simulink model "deadReckoningSim_soln"  (R2017a)
settings: Solver=FixedStepDiscrete  StartTime=0.0  StopTime=15  FixedStep=0.01  RelTol=1e-3
PreLoadFcn:
  | robotParameters;
values from neighbouring files (symbols this model uses):
  ticksPerRot = 627.2    [robotParameters.m]
  wheelR = 0.052    [robotParameters.m]
libraries: mobileRoboticsTrainingLib x3
settings Model: Creator=sseshadr  LastModifiedBy=shiremat

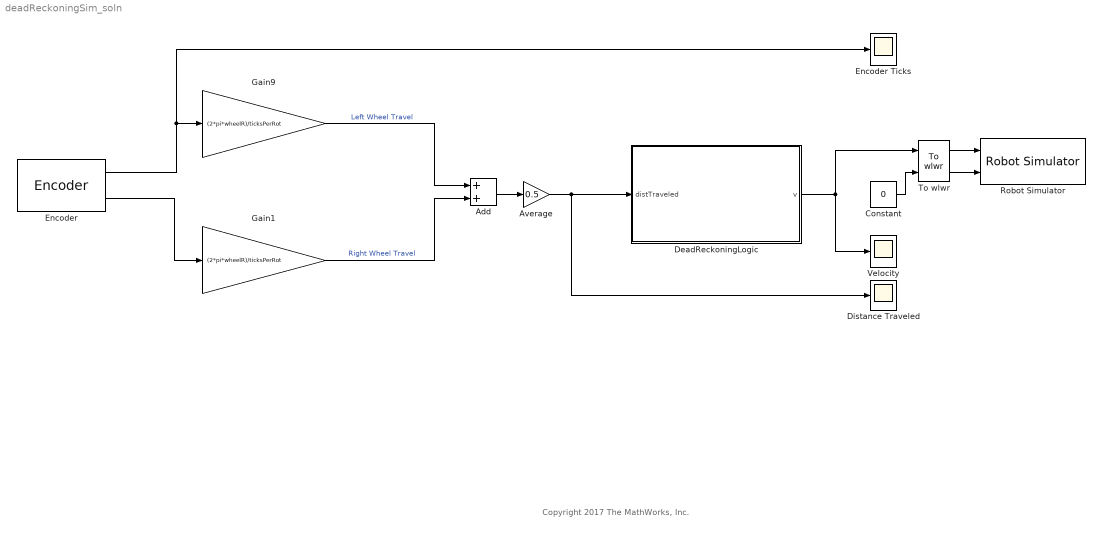
== system deadReckoningSim_soln ==
  note: Copyright 2017 The MathWorks, Inc.
  Add : Sum
  Average : Gain  Gain=0.5
  Constant : Constant  Value=0
  DeadReckoningLogic : Stateflow chart  TreatAsAtomicUnit=on
  Distance Traveled : Scope
  Encoder : mobileRoboticsTrainingLib/Encoder  axleLength=axleLength  wheelR=wheelR  ticksPerRot=ticksPerRot
      settings: SourceProductName=Mobile Robotics Training Library
  Encoder Ticks : Scope
  Gain1 : Gain  Gain=(2*pi*wheelR)/ticksPerRot
  Gain9 : Gain  Gain=(2*pi*wheelR)/ticksPerRot
  Robot Simulator : mobileRoboticsTrainingLib/Robot Simulator  Priority=99  mapVar=[]  startX=1  startY=1  startTheta=0  axleLength=axleLength  wheelR=wheelR
  To wlwr : mobileRoboticsTrainingLib/To wlwr  axleLength=axleLength  wheelR=wheelR
  Velocity : Scope
  wires:
  Average/1 -> DeadReckoningLogic/1(distTraveled), Distance Traveled/1
  DeadReckoningLogic/1(v) -> Velocity/1, To wlwr/1
  Gain9/1 -> Add/1  "Left Wheel Travel"
  Encoder/2 -> Gain1/1
  Encoder/1 -> Gain9/1, Encoder Ticks/1
  Add/1 -> Average/1
  Gain1/1 -> Add/2  "Right Wheel Travel"
  To wlwr/1 -> Robot Simulator/1
  To wlwr/2 -> Robot Simulator/2
  Constant/1 -> To wlwr/2

== stateflow chart deadReckoningSim_soln/DeadReckoningLogic ==
  state MoveForward
    entry:
    v = 0.1;
  state Stop
    entry:
    v = 0;
  (default) -> MoveForward : %Start Dead Reckoning
  MoveForward -> Stop : [distTraveled >= 1]
  data: v output; distTraveled input
